simulink model "PIDPPID"  (R2020a)
settings: Solver=VariableStepAuto  StartTime=0.0  StopTime=60  RelTol=1e-3
libraries: simulink x1
settings Model: Creator=axel_  LastModifiedBy=axel_

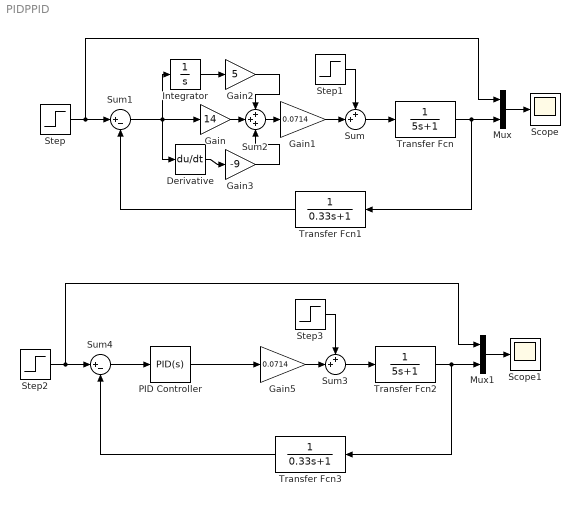
== system PIDPPID ==
  Derivative : Derivative
  Gain : Gain  Gain=14
  Gain1 : Gain  Gain=0.0714
  Gain2 : Gain  Gain=5
  Gain3 : Gain  Gain=-9
  Gain5 : Gain  Gain=0.0714
  Integrator : Integrator
  Mux : Mux  Inputs=2
  Mux1 : Mux  Inputs=2
  PID Controller : simulink/Continuous/PID Controller  Controller=PID  Form=Parallel  TimeDomain=Continuous-time  UseExternalTs=off  SampleTime=-1  IntegratorMethod=Forward Euler  FilterMethod=Forward Euler  ControllerParametersSource=internal  P=167.14652316933  I=79.8362115189374  D=54.5586819579116  UseFilter=on  N=246.940385069875  TunerSelectOption=Transfer Function Based (PID Tuner App)  InitialConditionSource=internal  InitialConditionForIntegrator=0  InitialConditionForFilter=0  DifferentiatorICPrevScaledInput=0  ExternalReset=none  TrackingMode=off  Kt=1  LimitOutput=off  UpperSaturationLimit=inf  LowerSaturationLimit=-inf  LinearizeAsGain=on  AntiWindupMode=none  Kb=1  POutMin=[]  POutMax=[]  IOutMin=[]  IOutMax=[]  DOutMin=[]  DOutMax=[]  NOutMin=[]  NOutMax=[]  SumOutMin=[]  SumOutMax=[]  SaturationOutMin=[]  SaturationOutMax=[]  PParamMin=[]  PParamMax=[]  IParamMin=[]  IParamMax=[]  DParamMin=[]  DParamMax=[]  NParamMin=[]  NParamMax=[]  KbParamMin=[]  KbParamMax=[]  KtParamMin=[]  KtParamMax=[]  KbOutMin=[]  KbOutMax=[]  KtOutMin=[]  KtOutMax=[]  IntegratorOutMin=[]  IntegratorOutMax=[]  FilterOutMin=[]  FilterOutMax=[]  SumI1OutMin=[]  SumI1OutMax=[]  SumI2OutMin=[]  SumI2OutMax=[]  SumI3OutMin=[]  SumI3OutMax=[]  SumI4OutMin=[]  SumI4OutMax=[]  SumDOutMin=[]  SumDOutMax=[]  DifferentiatorOutMin=[]  DifferentiatorOutMax=[]  FilterDiffOutCoefMin=[]  FilterDiffOutCoefMax=[]  ReciprocalOutMin=[]  ReciprocalOutMax=[]  SumDenOutMin=[]  SumDenOutMax=[]  SumNumOutMin=[]  SumNumOutMax=[]  DivideOutMin=[]  DivideOutMax=[]  UdiffTsProdOutMin=[]  UdiffTsProdOutMax=[]  NTsProdOutMin=[]  NTsProdOutMax=[]  UintegralTsProdOutMin=[]  UintegralTsProdOutMax=[]  UngainTsProdOutMin=[]  UngainTsProdOutMax=[]  IntegratorContinuousStateAttributes=''  IntegratorStateMustResolveToSignalObject=off  IntegratorRTWStateStorageClass=Auto  FilterContinuousStateAttributes=''  FilterStateMustResolveToSignalObject=off  FilterRTWStateStorageClass=Auto  ParallelPVariant=InternalParameters  IdealPVariant=Disabled  IVariant=InternalParameters  DVariant=InternalParameters  IntegratorVariant=Continuous  SatVariant=Disabled  AWVariant=Passthrough  PCopyVariant=Disabled  TRVariant=Disabled  FdbkBlocksVariant=Forward  IdealPFdbkVariant=Disabled  SatFdbkVariant=Disabled  DerivativeFilterVariant=ContFilter  NVariant=InternalParameters  NCopyVariant=Disabled  FilterICVariant=InternalICsFilter  IntegratorICVariant=InternalICs  ExternalResetVariant=Disabled  TRSumVariant=Passthrough  SumFdbkVariant=Disabled  SumVariant=Sum_PID  TsampFilterVariant=InternalTs  TsampNgainVariant=Passthrough  TsampIntegralVariant=Passthrough
  Scope : Scope
  Scope1 : Scope
  Step : Step  After=5  SampleTime=0.001
  Step1 : Step  After=0  SampleTime=0
  Step2 : Step  After=5  SampleTime=0.001
  Step3 : Step  After=0  SampleTime=0
  Sum : Sum  Inputs=++|
  Sum1 : Sum  Inputs=|+-
  Sum2 : Sum  Inputs=+++
  Sum3 : Sum  Inputs=++|
  Sum4 : Sum  Inputs=|+-
  Transfer Fcn : TransferFcn  Denominator=[5 1]
  Transfer Fcn1 : TransferFcn  Denominator=[0.33 1]
  Transfer Fcn2 : TransferFcn  Denominator=[5 1]
  Transfer Fcn3 : TransferFcn  Denominator=[0.33 1]
  wires:
  Sum/1 -> Transfer Fcn/1
  Gain1/1 -> Sum/2
  Mux/1 -> Scope/1
  Transfer Fcn/1 -> Transfer Fcn1/1, Mux/2
  Transfer Fcn1/1 -> Sum1/2
  Sum1/1 -> Derivative/1, Integrator/1, Gain/1
  Step/1 -> Mux/1, Sum1/1
  Step1/1 -> Sum/1
  Integrator/1 -> Gain2/1
  Gain2/1 -> Sum2/1
  Gain/1 -> Sum2/2
  Sum2/1 -> Gain1/1
  Derivative/1 -> Gain3/1
  Gain3/1 -> Sum2/3
  PID Controller/1 -> Gain5/1
  Step3/1 -> Sum3/1
  Step2/1 -> Sum4/1, Mux1/1
  Transfer Fcn3/1 -> Sum4/2
  Transfer Fcn2/1 -> Mux1/2, Transfer Fcn3/1
  Mux1/1 -> Scope1/1
  Gain5/1 -> Sum3/2
  Sum3/1 -> Transfer Fcn2/1
  Sum4/1 -> PID Controller/1
